simulink model "trail3"  (R2024a)
settings: Solver=VariableStepAuto  StartTime=0.0  StopTime=10.0  RelTol=1e-3
settings Model: Creator=DELL  LastModifiedBy=DELL

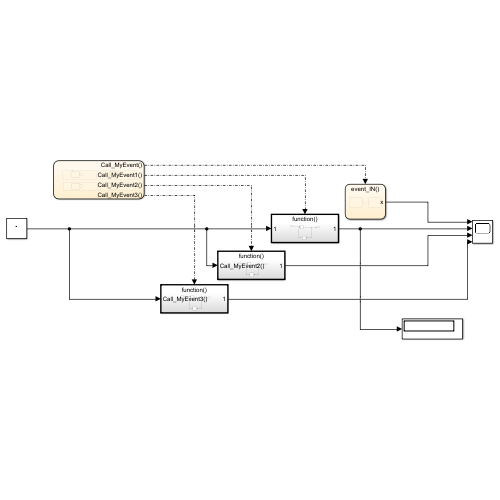
[thumbnail: Simulink's stored preview of the top-level diagram]
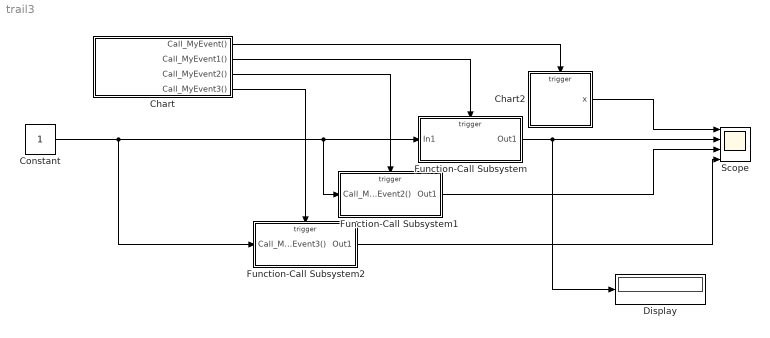
== system trail3 ==
  Chart : Stateflow chart  TreatAsAtomicUnit=on
  Chart2 : Stateflow chart  TreatAsAtomicUnit=on
  Constant : Constant  OutDataTypeStr=uint8
  Display : Display
      settings: Format=binary (Stored Integer)
  Function-Call Subsystem : Subsystem  TreatAsAtomicUnit=on
  Function-Call Subsystem1 : Subsystem  TreatAsAtomicUnit=on
  Function-Call Subsystem2 : Subsystem  TreatAsAtomicUnit=on
  Scope : Scope  NumInputPorts=4
  wires:
  Constant/1 -> Function-Call Subsystem2/1(Call_MyEvent3()), Function-Call Subsystem1/1(Call_MyEvent2()), Function-Call Subsystem/1(In1)
  Function-Call Subsystem/1(Out1) -> Display/1, Scope/2
  Chart/1(Call_MyEvent()) -> Chart2/Trigger
  Chart2/1(x) -> Scope/1
  Chart/2(Call_MyEvent1()) -> Function-Call Subsystem/Trigger
  Chart/3(Call_MyEvent2()) -> Function-Call Subsystem1/Trigger
  Chart/4(Call_MyEvent3()) -> Function-Call Subsystem2/Trigger
  Function-Call Subsystem1/1(Out1) -> Scope/3
  Function-Call Subsystem2/1(Out1) -> Scope/4

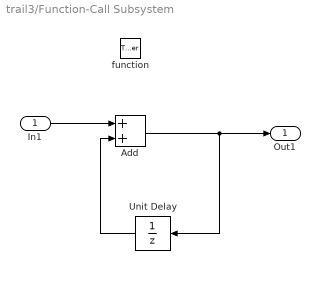
== system trail3/Function-Call Subsystem ==
  In1 : Inport
  function : TriggerPort  TriggerType=function-call  VariantControl=(inherit)
  Add : Sum
  Unit Delay : UnitDelay  SampleTime=-1  HasFrameUpgradeWarning=on
  Out1 : Outport
  wires:
  In1/1 -> Add/1
  Unit Delay/1 -> Add/2
  Add/1 -> Unit Delay/1, Out1/1

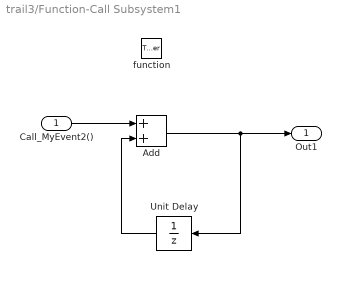
== system trail3/Function-Call Subsystem1 ==
  Call_MyEvent2() : Inport
  function : TriggerPort  TriggerType=function-call  VariantControl=(inherit)
  Add : Sum
  Unit Delay : UnitDelay  SampleTime=-1  HasFrameUpgradeWarning=on
  Out1 : Outport
  wires:
  Add/1 -> Out1/1, Unit Delay/1
  Unit Delay/1 -> Add/2
  Call_MyEvent2()/1 -> Add/1

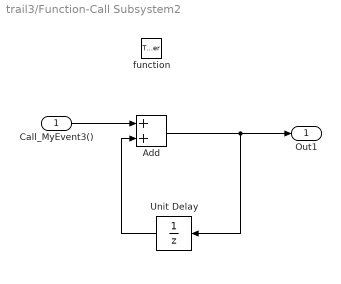
== system trail3/Function-Call Subsystem2 ==
  Call_MyEvent3() : Inport
  function : TriggerPort  TriggerType=function-call  VariantControl=(inherit)
  Add : Sum
  Unit Delay : UnitDelay  SampleTime=-1  HasFrameUpgradeWarning=on
  Out1 : Outport
  wires:
  Call_MyEvent3()/1 -> Add/1
  Unit Delay/1 -> Add/2
  Add/1 -> Unit Delay/1, Out1/1

== stateflow chart trail3/Chart2 ==
  state State_A
    en:
    x=3;
  state State_B
    en:
    x=6;
  (default) -> State_A
  State_A -> State_B : event_IN
  State_B -> State_A : event_IN
  data: x output
  events: event_IN input FUNCTION_CALL_EVENT

== stateflow chart trail3/Chart ==
  state State_A [parallel]
    settings: executionOrder=1
    state A
    State_A.A -> State_A.A : after(0.5,sec)/{Call_MyEvent}
  state State_C [parallel]
    settings: executionOrder=3
    state A
    State_C.A -> State_C.A : after(1.5,sec)/{Call_MyEvent2}
  state State_B [parallel]
    settings: executionOrder=2
    state B
    State_B.B -> State_B.B : after(1,sec)/{Call_MyEvent1}
  state State_D [parallel]
    settings: executionOrder=4
    state B
    State_D.B -> State_D.B : after(2  ,sec)/{Call_MyEvent3}
  (default) -> State_A.A [order 1]
  (default) -> State_C.A [order 2]
  events: Call_MyEvent output FUNCTION_CALL_EVENT; Call_MyEvent1 output FUNCTION_CALL_EVENT; Call_MyEvent2 output FUNCTION_CALL_EVENT; Call_MyEvent3 output FUNCTION_CALL_EVENT
